simulink model "aeroblk_self_cond_cntr"  (Simulink 6.0)
settings: Solver=ode45  StartTime=0.0  StopTime=10.0  RelTol=1e-3
libraries: aerolibschedule x1
settings Model: Creator=The MathWorks Inc.  LastModifiedBy=batserve  ExtModeAutoUpdateStatusClock=off
settings OptimizationCC: BooleanDataType=off
settings DebuggingCC: CheckExecutionContextPreStartOutputMsg=on  CheckExecutionContextRuntimeOutputMsg=on  SolverPrmCheckMsg=none
settings HardwareCC: TargetUnknown=on

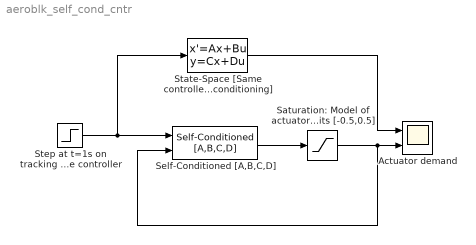
== system aeroblk_self_cond_cntr ==
  Actuator demand : Scope  NumInputPorts=2
      settings: YMin=-1~-0.2  YMax=9~0.8
  Saturation: Model of actuator authority limits [-0.5,0.5] : Saturate
  Self-Conditioned [A,B,C,D] : aerolibschedule/Self-Conditioned [A,B,C,D]  Ak=[0 -0.2;0 -3]  Bk=[1;1]  Ck=[1 0]  Dk=0.02  x_initial=0  vec_w=[-5 -2]
  "State-Space [Same controller, no self conditioning]" : StateSpace  A=[0 -0.2;0 -3]  B=[1;1]  C=[1 0]  D=0.02
  Step at t=1s on tracking error sent to the controller : Step  SampleTime=0
  wires:
  Self-Conditioned [A,B,C,D]/1 -> Saturation: Model of actuator authority limits [-0.5,0.5]/1
  Step at t=1s on tracking error sent to the controller/1 -> Self-Conditioned [A,B,C,D]/1, "State-Space [Same controller, no self conditioning]"/1
  Saturation: Model of actuator authority limits [-0.5,0.5]/1 -> Self-Conditioned [A,B,C,D]/2, Actuator demand/2
  "State-Space [Same controller, no self conditioning]"/1 -> Actuator demand/1
